simulink model "PART_5_COMBINED_HWY"  (R2025a)
settings: Solver=ode4  StartTime=0.0  StopTime=763  RelTol=1e-3
values from neighbouring files (symbols this model uses):
  Air_density = 1.225    [PART_5_CITY.m]    (also in PART_5_HWY.m; PART_5_SCO3.m; PART_5_US06_MODEL.m)
  Coefficient_of_rolling_resistance = 0.012    [PART_5_CITY.m]    (also in PART_5_HWY.m; PART_5_SCO3.m; PART_5_US06_MODEL.m)
  Drag_coefficient = 0.2    [PART_5_CITY.m]    (also in PART_5_HWY.m; PART_5_SCO3.m; PART_5_US06_MODEL.m)
  Driveline_model_spinloss = 6    [PART_5_CITY.m]    (also in PART_5_HWY.m; PART_5_SCO3.m; PART_5_US06_MODEL.m)
  energy_capacity = 12.6    [PART_5_CITY.m]    (also in PART_5_HWY.m; PART_5_SCO3.m; PART_5_US06_MODEL.m)
  Frontal_Area = 1.8    [PART_5_CITY.m]    (also in PART_5_HWY.m; PART_5_SCO3.m; PART_5_US06_MODEL.m)
  Gear_Ratio_g = 7    [PART_5_CITY.m]    (also in PART_5_HWY.m; PART_5_SCO3.m; PART_5_US06_MODEL.m)
  grade_angle = 15    [PART_5_CITY.m]    (also in PART_5_HWY.m; PART_5_SCO3.m; PART_5_US06_MODEL.m)
  Gravitational_force = 9.81    [PART_5_CITY.m]    (also in PART_5_HWY.m; PART_5_SCO3.m; PART_5_US06_MODEL.m)
  initial_soc = 0.95    [PART_5_CITY.m]    (also in PART_5_HWY.m; PART_5_SCO3.m; PART_5_US06_MODEL.m)
  MDL_brakesystem_friction = 0.45    [PART_5_CITY.m]    (also in PART_5_HWY.m; PART_5_SCO3.m; PART_5_US06_MODEL.m)
  MDL_brakesystem_regenerative_friction = 0.55    [PART_5_CITY.m]    (also in PART_5_HWY.m; PART_5_SCO3.m; PART_5_US06_MODEL.m)
  MDL_Brakingsystem_maximum_brakeforce = 10000    [PART_5_CITY.m]    (also in PART_5_HWY.m; PART_5_SCO3.m; PART_5_US06_MODEL.m)
  MDL_motormodel_Kc = 0.045257    [PART_5_CITY.m]    (also in PART_5_HWY.m; PART_5_SCO3.m; PART_5_US06_MODEL.m)
  MDL_motormodel_max_power_out = 100000    [PART_5_CITY.m]    (also in PART_5_HWY.m; PART_5_SCO3.m; PART_5_US06_MODEL.m)
  MDL_motormodel_maxtorque_out = 500    [PART_5_CITY.m]    (also in PART_5_HWY.m; PART_5_SCO3.m; PART_5_US06_MODEL.m)
  MotorModel_C = 628.3    [PART_5_CITY.m]    (also in PART_5_HWY.m; PART_5_SCO3.m; PART_5_US06_MODEL.m)
  MotorModel_ki = 0.016667    [PART_5_CITY.m]    (also in PART_5_HWY.m; PART_5_SCO3.m; PART_5_US06_MODEL.m)
  MotorModel_kw = 5.0664*10^-5    (= 5.0664e-05)    [PART_5_CITY.m]    (also in PART_5_HWY.m; PART_5_SCO3.m; PART_5_US06_MODEL.m)
  total_weight = 2154.6    [PART_5_CITY.m]    (also in PART_5_HWY.m; PART_5_SCO3.m; PART_5_US06_MODEL.m)
  wheel_radius_cal = 0.217    [PART_5_CITY.m]    (also in PART_5_HWY.m; PART_5_SCO3.m; PART_5_US06_MODEL.m)
undefined symbols (not defined in the file or in its folder): m, magnitude, s
libraries: simulink x5, aerolibconvert2 x4, slpidlib x1
settings Model: Creator=user  LastModifiedBy=user

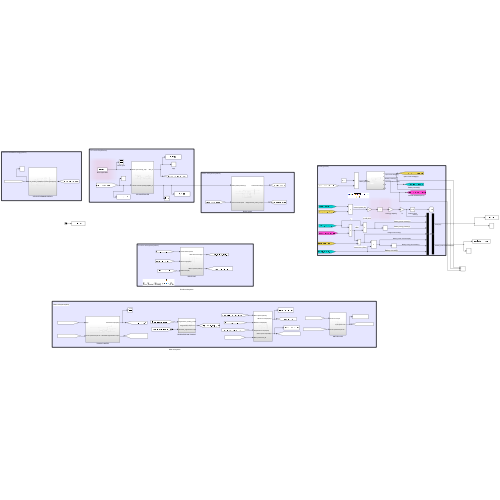
[thumbnail: Simulink's stored preview of the top-level diagram]
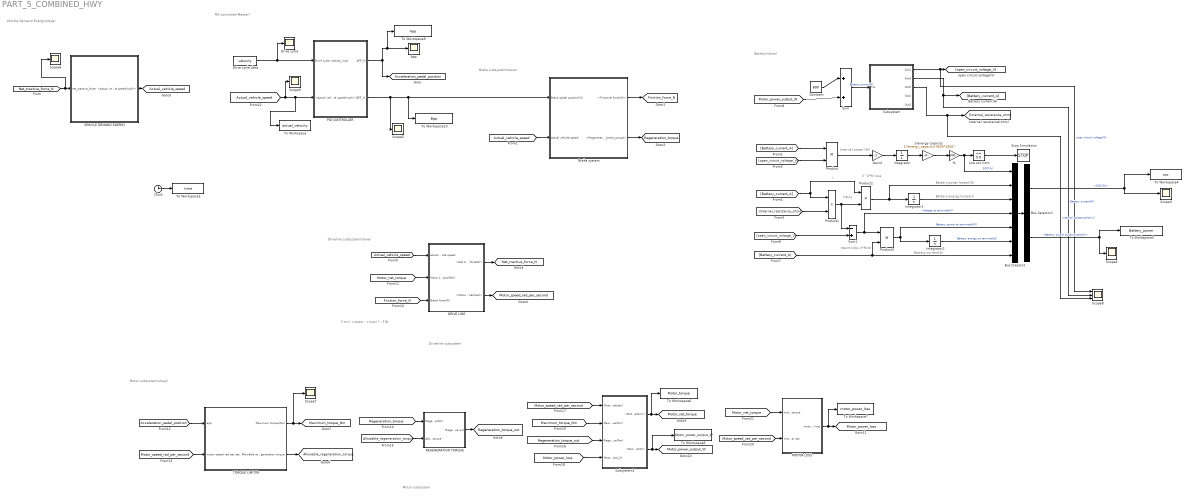
== system PART_5_COMBINED_HWY ==
  note: F tr=( τ motor - τ loss) * - F Br
  note: PID controller(Master)
  note: Driveline subsystem
  note: Vehicle Demand Energy(slave)
  note: Motor subsystem
  note: Driveline subsystem(slave)
  note: Brake subsystem(slave)
  note: Battery energy losses(J)
  note: (I^2*R) loss
  note: Battery power losses(W)
  note: Battery(slave)
  note: I*Rint
  note: Battery current(A)
  note: Internal power (W)
  note: I
  note: Motor subsystem(slave)
  note: Vterm=Voc-(I*Rint)
  % : Gain  Gain=100
  1/energy capacity : Gain  Gain=1/(energy_capacity*3600*1000)
  App : Scope
      settings: ActiveDisplayYMinimum=-0.92182  ActiveDisplayYMaximum=8.29642
  Brake system : Subsystem
  Bus Creator2 : BusCreator  Inputs=7
  Bus Selector1 : BusSelector  OutputSignals=SOC(%),Battery power at terminals(W)
  Clock : Clock
  Constant : Constant  Value=600
  DRIVE LINE : Subsystem
  Drive cycle : Scope
      settings: ActiveDisplayYMinimum=-10.0375  ActiveDisplayYMaximum=90.3375  DataLoggingVariableName=ScopeData12
  Drive cycle data : FromWorkspace  VariableName=velocity  SampleTime=0.1
  Gain4 : Gain  Gain=-1
  Integrator : Integrator  InitialCondition=energy_capacity*3600*1000*initial_soc
  Integrator1 : Integrator
  Integrator2 : Integrator
  Low soc limit : simulink/Logic and Bit Operations/Compare To Constant  relop=<=  const=5.0  OutDataTypeStr=boolean
  MOTOR LOSS : Subsystem
  PID CONTROLLER : Subsystem
  Product{,1..3} (4 alike) : Product
  REGENERATION TORQUE : Subsystem
  Scope{3..7,9} (6 alike) : Scope
      Scope3 settings: ActiveDisplayYMinimum=-1  ActiveDisplayYMaximum=1  DataLoggingVariableName=ScopeData13
      Scope4 settings: ActiveDisplayYMinimum=-68149.999999999942  ActiveDisplayYMaximum=119350.00000000003  DataLoggingVariableName=ScopeData14
      Scope5 settings: ActiveDisplayYMinimum=-1  ActiveDisplayYMaximum=1  DataLoggingVariableName=ScopeData6
      Scope6 settings: ActiveDisplayYMinimum=-11875  ActiveDisplayYMaximum=6875  DataLoggingVariableName=ScopeData15
      Scope7 settings: ActiveDisplayYMinimum=-1  ActiveDisplayYMaximum=1  DataLoggingVariableName=ScopeData16
      Scope9 settings: ActiveDisplayYMinimum=-1  ActiveDisplayYMaximum=1  DataLoggingVariableName=ScopeData17
  Scope8 : Scope  NumInputPorts=3
      settings: ActiveDisplayYMinimum=-1  ActiveDisplayYMaximum=1  DataLoggingVariableName=ScopeData9
  Stop Simulation : Stop
  Subsystem : Subsystem
  Subsystem1 : Subsystem
  Sum : Sum  Inputs=|++
  Sum1 : Sum  Inputs=-+
  TORQUE LIMITER : Subsystem
  To Workspace : ToWorkspace  VariableName=actual_velocity  SampleTime=-1
      settings: Save2DSignal=2-D array (concatenate along first dimension)
  To Workspace1 : ToWorkspace  VariableName=time  SampleTime=-1
      settings: Save2DSignal=2-D array (concatenate along first dimension)
  To Workspace10 : ToWorkspace  VariableName=Bpp  SampleTime=-1
      settings: Save2DSignal=2-D array (concatenate along first dimension)
  To Workspace4 : ToWorkspace  VariableName=soc  SampleTime=-1
      settings: Save2DSignal=2-D array (concatenate along first dimension)
  To Workspace5 : ToWorkspace  VariableName=Battery_power  SampleTime=-1
      settings: Save2DSignal=2-D array (concatenate along first dimension)
  To Workspace6 : ToWorkspace  VariableName=Motor_torque  SampleTime=-1
      settings: Save2DSignal=2-D array (concatenate along first dimension)
  To Workspace7 : ToWorkspace  VariableName=motor_power_loss  SampleTime=-1
      settings: Save2DSignal=2-D array (concatenate along first dimension)
  To Workspace8 : ToWorkspace  VariableName=Motor_power_output_W  SampleTime=-1
      settings: Save2DSignal=2-D array (concatenate along first dimension)
  To Workspace9 : ToWorkspace  VariableName=App  SampleTime=-1
      settings: Save2DSignal=2-D array (concatenate along first dimension)
  VEHICLE DEMAND ENERGY : Subsystem
  tag scope: Acceleration_pedal_position=global, Actual_vehicle_speed=global, Allowable_regeneration_torque=global, Friction_force_N=global, Maximum_torque_Nm=global, Motor_net_torque=global, Motor_power_loss=global, Motor_power_output_W=global, Motor_speed_rad_per_second=global, Net_tractive_force_N=global, Regeneration_torque=global, Regeneration_torque_out=global
  wires:
  [Internal_resistance_ohm] -> Product1/2
  Integrator2/1 -> Bus Creator2/6  "Battery energy at terminals(J)"
  Subsystem/2(Out4) -> Scope8/2, [Battery_current_A]  "Battery current(A)"
  [Maximum_torque_Nm] -> Subsystem1/2(Maximum torque(Nm))
  [Battery_current_A] -> Product/1
  DRIVE LINE/2(<Motor speed (rad/sec)>) -> [Motor_speed_rad_per_second]
  [Friction_force_N] -> DRIVE LINE/3(Brake force(N))
  [Motor_net_torque] -> MOTOR LOSS/1(motor net torque)
  %/1 -> Bus Creator2/1, Low soc limit/1  "SOC(%)"
  Subsystem/3(Out5) -> Scope8/3, [Internal_resistance_ohm]  "Internal resistance(ohm)"
  Drive cycle data/1 -> Drive cycle/1, PID CONTROLLER/1(Drive cycle velocity_mph)
  Subsystem/1(Out1) -> Scope8/1, [open_circuit_voltage_V]  "open circuit voltage(V)"
  Subsystem1/1(<Motor net torque(Nm)>) -> To Workspace6/1, [Motor_net_torque]
  [Actual_vehicle_speed] -> DRIVE LINE/1(actual vehicle speed)
  [Motor_power_output_W] -> Sum/2
  Bus Selector1/1 -> To Workspace4/1, Scope3/1  "<SOC(%)>"
  [Net_tractive_force_N] -> Scope6/1, VEHICLE DEMAND ENERGY/1(net_tractive_force)
  Product/1 -> Gain4/1
  Low soc limit/1 -> Stop Simulation/1
  [Motor_speed_rad_per_second] -> Subsystem1/1(Motor speed (rad/sec))
  DRIVE LINE/1(<Net tractive force(N)>) -> [Net_tractive_force_N]
  [Motor_speed_rad_per_second] -> MOTOR LOSS/2(motor speed rad per sec)
  Sum/1 -> Subsystem/1(In1)  "Battery power(W)"
  [Regeneration_torque] -> REGENERATION TORQUE/1(Regeneration_braking_torque(Nm))
  Product3/1 -> Integrator2/1, Bus Creator2/5  "Battery power at terminals(W)"
  Product1/1 -> Sum1/1, Product2/2
  [Actual_vehicle_speed] -> Scope9/1, To Workspace/1, PID CONTROLLER/2(<Actual vehicle speed(mph)>)
  Brake system/2(<Regenerative_brake_torque>) -> [Regeneration_torque]
  REGENERATION TORQUE/1(Regeneration torque out) -> [Regeneration_torque_out]
  [Motor_net_torque] -> DRIVE LINE/2(Motor torque(Nm))
  Subsystem1/2(<Motor power output(W)>) -> To Workspace8/1, [Motor_power_output_W]
  [Regeneration_torque_out] -> Subsystem1/3(Regeneration torque(Nm))
  Integrator/1 -> 1/energy capacity/1
  [Allowable_regeneration_torque] -> REGENERATION TORQUE/2(Allowable_regeneration torque)
  [Battery_current_A] -> Product3/2, Bus Creator2/7
  [Motor_speed_rad_per_second] -> TORQUE LIMITER/2(motor speed rad per sec)
  Sum1/1 -> Product3/1, Bus Creator2/4  "Voltage at terminals(V)"
  MOTOR LOSS/1(motor power loss) -> To Workspace7/1, [Motor_power_loss]
  [Acceleration_pedal_position] -> TORQUE LIMITER/1(app)
  PID CONTROLLER/2(BPP_%) -> To Workspace10/1, Brake system/1(Brake pedal position(%)), Scope5/1
  Brake system/1(<Frictional force(N)>) -> [Friction_force_N]
  PID CONTROLLER/1(APP_%) -> To Workspace9/1, App/1, [Acceleration_pedal_position]
  Product2/1 -> Bus Creator2/2, Integrator1/1
  Bus Selector1/2 -> Scope4/1, To Workspace5/1  "<Battery power at terminals(W)>"
  Integrator1/1 -> Bus Creator2/3
  [Motor_power_loss] -> Subsystem1/4(Motor power loss_W)
  TORQUE LIMITER/1(Maximum torque(Nm)) -> Scope7/1, [Maximum_torque_Nm]
  1/energy capacity/1 -> %/1
  Constant/1 -> Sum/1
  TORQUE LIMITER/2(Allowable regeneration torque) -> [Allowable_regeneration_torque]
  [open_circuit_voltage_V] -> Sum1/2
  Gain4/1 -> Integrator/1
  Clock/1 -> To Workspace1/1
  Bus Creator2/1 -> Bus Selector1/1
  VEHICLE DEMAND ENERGY/1(<Actual vehicle speed(mph)>) -> [Actual_vehicle_speed]
  [open_circuit_voltage_V] -> Product/2
  [Actual_vehicle_speed] -> Brake system/2(Actual vehicle speed)
  [Battery_current_A] -> Product2/1, Product1/1

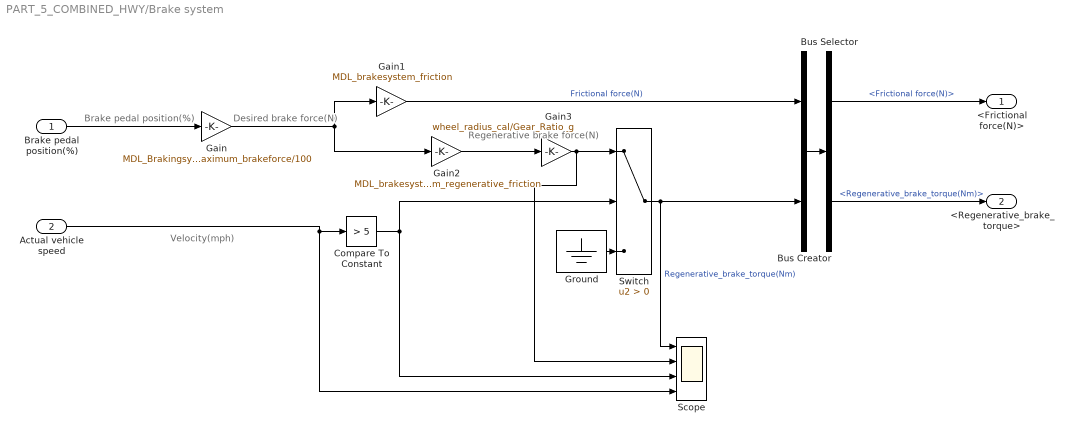
== system PART_5_COMBINED_HWY/Brake system ==
  note: Desired brake force(N)
  note: Brake pedal position(%)
  note: Velocity(mph)
  note: Regenerative
      | brake force(N)
  Brake pedal position(%) : Inport
  Actual vehicle speed : Inport  Port=2
  Bus Creator : BusCreator  Inputs=2
  Bus Selector : BusSelector  OutputSignals=Frictional force(N),Regenerative_brake_torque(Nm)
  Compare To Constant : simulink/Logic and Bit Operations/Compare To Constant  relop=>  const=5  OutDataTypeStr=boolean
  Gain : Gain  Gain=MDL_Brakingsystem_maximum_brakeforce/100
  Gain1 : Gain  Gain=MDL_brakesystem_friction
  Gain2 : Gain  Gain=MDL_brakesystem_regenerative_friction
  Gain3 : Gain  Gain=wheel_radius_cal/Gear_Ratio_g
  Ground : Ground
  Scope : Scope  NumInputPorts=4
      settings: ActiveDisplayYMinimum=-1  ActiveDisplayYMaximum=1  DataLoggingVariableName=ScopeData3
  Switch : Switch  Criteria=u2 > Threshold  SaturateOnIntegerOverflow=off  InputSameDT=off
  <Frictional force(N)> : Outport
  <Regenerative_brake_torque> : Outport  Port=2
  wires:
  Gain2/1 -> Gain3/1
  Switch/1 -> Bus Creator/2, Scope/1  "Regenerative_brake_torque(Nm)"
  Bus Creator/1 -> Bus Selector/1
  Gain1/1 -> Bus Creator/1  "Frictional force(N)"
  Compare To Constant/1 -> Scope/3, Switch/2
  Gain3/1 -> Scope/2, Switch/1
  Ground/1 -> Switch/3
  Gain/1 -> Gain2/1, Gain1/1
  Actual vehicle speed/1 -> Scope/4, Compare To Constant/1
  Bus Selector/2 -> <Regenerative_brake_torque>/1  "<Regenerative_brake_torque(Nm)>"
  Brake pedal position(%)/1 -> Gain/1
  Bus Selector/1 -> <Frictional force(N)>/1  "<Frictional force(N)>"

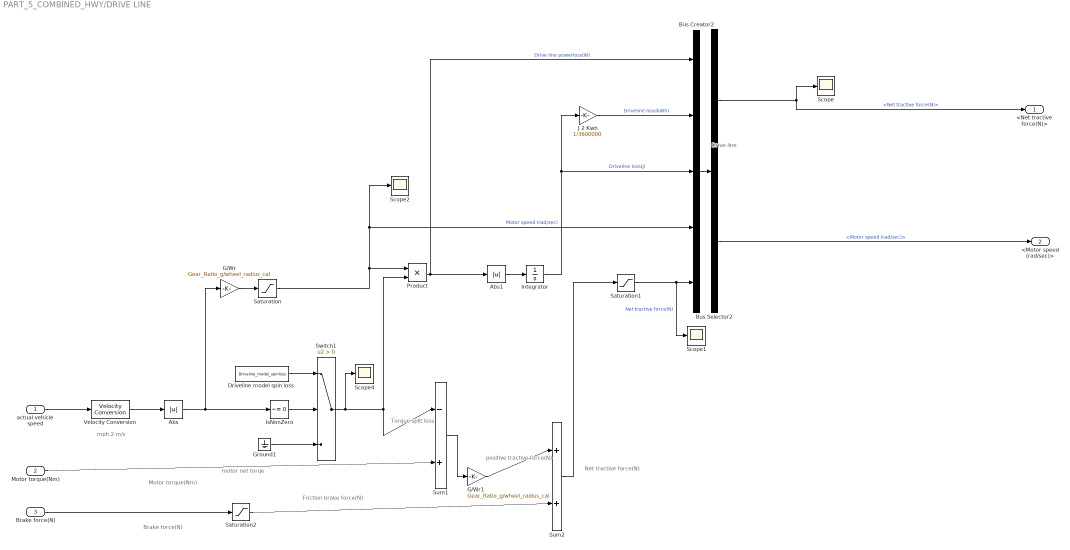
== system PART_5_COMBINED_HWY/DRIVE LINE ==
  note: Drive line
  note: Friction brake force(N)
  note: Net tractive force(N)
  note: motor net torqe
  note: positive tractive force(N)
  note: mph 2 m/s
  note: Motor torque(Nm)
  note: Torque split
      |  loss
  note: Brake force(N)
  actual vehicle speed : Inport
  Motor torque(Nm) : Inport  Port=2
  Brake force(N) : Inport  Port=3
  Abs : Abs  SaturateOnIntegerOverflow=off
  Abs1 : Abs  SaturateOnIntegerOverflow=off
  Bus Creator2 : BusCreator  Inputs=5
  Bus Selector2 : BusSelector  OutputSignals=Net tractive force(N),Motor speed (rad/sec)
  Driveline model spin loss : Constant  Value=Driveline_model_spinloss  OutDataTypeStr=double
  G/Wr : Gain  Gain=Gear_Ratio_g/wheel_radius_cal
  G/Wr1 : Gain  Gain=Gear_Ratio_g/wheel_radius_cal
  Ground1 : Ground
  Integrator : Integrator
  IsNonZero : simulink/Logic and Bit Operations/Compare To Zero  relop=~=  OutDataTypeStr=boolean
  J 2 Kwh : Gain  Gain=1/3600000
  Product : Product
  Saturation : Saturate  UpperLimit=inf  LowerLimit=.00001
  Saturation1 : Saturate  UpperLimit=5000  LowerLimit=-10000  OutDataTypeStr=double
  Saturation2 : Saturate  UpperLimit=0  LowerLimit=-10000
  Scope{,1..2,4} (4 alike) : Scope
      Scope settings: ActiveDisplayYMinimum=-1  ActiveDisplayYMaximum=1
      Scope1 settings: ActiveDisplayYMinimum=-10214.22916  ActiveDisplayYMaximum=10023.80324  DataLoggingVariableName=ScopeData3
      Scope2 settings: ActiveDisplayYMinimum=-7.75811  ActiveDisplayYMaximum=69.82309  DataLoggingVariableName=ScopeData4
      Scope4 settings: ActiveDisplayYMinimum=-0.75  ActiveDisplayYMaximum=6.75  DataLoggingVariableName=ScopeData11
  Sum1 : Sum  Inputs=|-+
  Sum2 : Sum  Inputs=|++
  Switch1 : Switch  Criteria=u2 > Threshold  OutDataTypeStr=double  SaturateOnIntegerOverflow=off  InputSameDT=off
  Velocity Conversion : aerolibconvert2/Velocity Conversion  IU=mph  OU=m/s
  <Net tractive force(N)> : Outport
  <Motor speed (rad/sec)> : Outport  Port=2
  wires:
  Abs/1 -> IsNonZero/1, G/Wr/1
  Saturation/1 -> Bus Creator2/4, Scope2/1, Product/1  "Motor speed (rad/sec)"
  Abs1/1 -> Integrator/1
  Switch1/1 -> Product/2, Sum1/1, Scope4/1
  Sum2/1 -> Saturation1/1
  Ground1/1 -> Switch1/3
  Sum1/1 -> G/Wr1/1
  G/Wr1/1 -> Sum2/1
  Saturation1/1 -> Scope1/1, Bus Creator2/5  "Net tractive force(N)"
  Product/1 -> Bus Creator2/1, Abs1/1  "Drive line powerloss(W)"
  Integrator/1 -> J 2 Kwh/1, Bus Creator2/3  "Driveline loss(J)"
  G/Wr/1 -> Saturation/1
  J 2 Kwh/1 -> Bus Creator2/2  "Driveline loss(kWh)"
  actual vehicle speed/1 -> Velocity Conversion/1
  Bus Selector2/2 -> <Motor speed (rad/sec)>/1  "<Motor speed (rad/sec)>"
  IsNonZero/1 -> Switch1/2
  Velocity Conversion/1 -> Abs/1
  Bus Creator2/1 -> Bus Selector2/1
  Saturation2/1 -> Sum2/2
  Motor torque(Nm)/1 -> Sum1/2
  Bus Selector2/1 -> Scope/1, <Net tractive force(N)>/1  "<Net tractive force(N)>"
  Brake force(N)/1 -> Saturation2/1
  Driveline model spin loss/1 -> Switch1/1

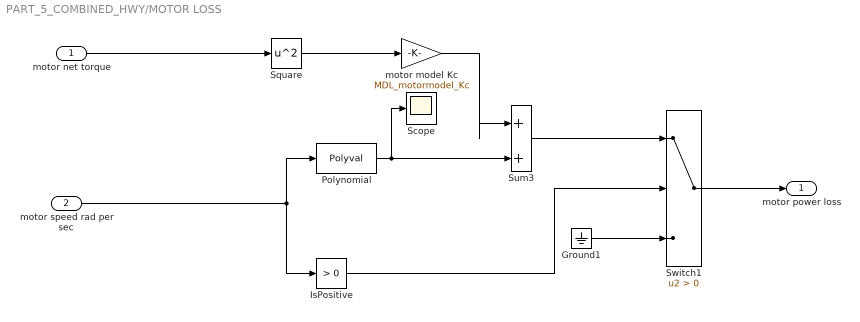
== system PART_5_COMBINED_HWY/MOTOR LOSS ==
  motor net torque : Inport
  motor speed rad per sec : Inport  Port=2
  Ground1 : Ground
  IsPositive : simulink/Logic and Bit Operations/Compare To Zero  relop=>  OutDataTypeStr=boolean
  Polynomial : Polyval  Coefs=[MotorModel_kw,0,MotorModel_ki,MotorModel_C]
  Scope : Scope
      settings: ActiveDisplayYMinimum=583.90938  ActiveDisplayYMaximum=1027.81559  DataLoggingVariableName=ScopeData5
  Square : Math  Operator=square
  Sum3 : Sum  Inputs=|++
  Switch1 : Switch  Criteria=u2 > Threshold  OutDataTypeStr=double  SaturateOnIntegerOverflow=off  InputSameDT=off
  motor model Kc : Gain  Gain=MDL_motormodel_Kc
  motor power loss : Outport
  wires:
  Polynomial/1 -> Scope/1, Sum3/2
  Sum3/1 -> Switch1/1
  Square/1 -> motor model Kc/1
  Ground1/1 -> Switch1/3
  motor model Kc/1 -> Sum3/1
  IsPositive/1 -> Switch1/2
  Switch1/1 -> motor power loss/1
  motor net torque/1 -> Square/1
  motor speed rad per sec/1 -> Polynomial/1, IsPositive/1

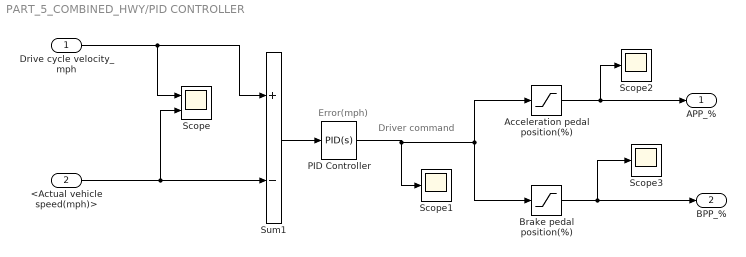
== system PART_5_COMBINED_HWY/PID CONTROLLER ==
  note: Driver command
  note: Error(mph)
  Drive cycle velocity_mph : Inport
  <Actual vehicle speed(mph)> : Inport  Port=2
  Acceleration pedal position(%) : Saturate  UpperLimit=100  LowerLimit=0  LinearizeAsGain=off  ZeroCross=off  OutDataTypeStr=double
  Brake pedal position(%) : Saturate  UpperLimit=0  LowerLimit=-100  LinearizeAsGain=off  ZeroCross=off  OutDataTypeStr=double
  PID Controller : slpidlib/PID Controller  Controller=PID  Form=Parallel  TimeDomain=Continuous-time  UseExternalTs=off  SampleTime=-1  IntegratorMethod=Forward Euler  FilterMethod=Forward Euler  ControllerParametersSource=internal  P=250  I=50  UseKiTs=off  D=0  UseExternalDerivativeSource=off  N=10  UseFilter=on  TunerSelectOption=Transfer Function Based (PID Tuner App)  InitialConditionSource=internal  InitialConditionForIntegrator=0  InitialConditionForFilter=0  DifferentiatorICPrevScaledInput=0  ExternalReset=none  TrackingMode=off  Kt=1  LimitOutput=off  SatLimitsSource=internal  UpperSaturationLimit=inf  LowerSaturationLimit=-inf  LinearizeAsGain=off  AntiWindupMode=none  Kb=1  LimitIntegrator=off  UpperIntegratorSaturationLimit=inf  LowerIntegratorSaturationLimit=-inf  POutMin=[]  POutMax=[]  IOutMin=[]  IOutMax=[]  DOutMin=[]  DOutMax=[]  NOutMin=[]  NOutMax=[]  SumOutMin=[]  SumOutMax=[]  SaturationOutMin=[]  SaturationOutMax=[]  PParamMin=[]  PParamMax=[]  IParamMin=[]  IParamMax=[]  DParamMin=[]  DParamMax=[]  NParamMin=[]  NParamMax=[]  KbParamMin=[]  KbParamMax=[]  KtParamMin=[]  KtParamMax=[]  KbOutMin=[]  KbOutMax=[]  KtOutMin=[]  KtOutMax=[]  IntegratorOutMin=[]  IntegratorOutMax=[]  FilterOutMin=[]  FilterOutMax=[]  SumI1OutMin=[]  SumI1OutMax=[]  SumI2OutMin=[]  SumI2OutMax=[]  SumI3OutMin=[]  SumI3OutMax=[]  SumI4OutMin=[]  SumI4OutMax=[]  SumDOutMin=[]  SumDOutMax=[]  DifferentiatorOutMin=[]  DifferentiatorOutMax=[]  FilterDiffOutCoefMin=[]  FilterDiffOutCoefMax=[]  ReciprocalOutMin=[]  ReciprocalOutMax=[]  SumDenOutMin=[]  SumDenOutMax=[]  SumNumOutMin=[]  SumNumOutMax=[]  DivideOutMin=[]  DivideOutMax=[]  UdiffTsProdOutMin=[]  UdiffTsProdOutMax=[]  NTsProdOutMin=[]  NTsProdOutMax=[]  UintegralTsProdOutMin=[]  UintegralTsProdOutMax=[]  UngainTsProdOutMin=[]  UngainTsProdOutMax=[]  ClampingZeroOutDataTypeStr=Inherit: Inherit via back propagation  ClampingZeroOutMin=[]  ClampingZeroOutMax=[]  FilterDenConstantOutDataTypeStr=Inherit: Inherit via back propagation  FilterDenConstantOutMin=[]  FilterDenConstantOutMax=[]  PCopyOutDataTypeStr=Inherit: Inherit via back propagation  PCopyOutMin=[]  PCopyOutMax=[]  NCopyOutDataTypeStr=Inherit: Inherit via back propagation  NCopyOutMin=[]  NCopyOutMax=[]  IntegratorContinuousStateAttributes=''  IntegratorStateMustResolveToSignalObject=off  IntegratorRTWStateStorageClass=Auto  FilterContinuousStateAttributes=''  FilterStateMustResolveToSignalObject=off  FilterRTWStateStorageClass=Auto  ParallelPVariant=InternalParameters  IdealPVariant=Disabled  IVariant=InternalParameters  DVariant=InternalParameters  IntegratorVariant=Continuous  SatVariant=Disabled  AWVariant=Passthrough  PCopyVariant=Disabled  TRVariant=Disabled  FdbkBlocksVariant=Forward  IdealPFdbkVariant=Disabled  SatFdbkVariant=Disabled  DerivativeFilterVariant=ContFilter  NVariant=InternalParameters  NCopyVariant=Disabled  FilterICVariant=InternalICsFilter  IntegratorICVariant=InternalICs  ExternalResetVariant=Disabled  TRSumVariant=Passthrough  SumFdbkVariant=Disabled  SumVariant=Sum_PID  TsampFilterVariant=InternalTs  TsampNgainVariant=Passthrough  TsampIntegralVariant=Disabled_SignalSpec  ExternalSaturationOutDataTypeStr=Inherit: Same as second input  DerivativeSourceVariant=ErrorSignal  PreIntVariant=InternalPreInt
  Scope : Scope  NumInputPorts=2
      settings: ActiveDisplayYMinimum=-1  ActiveDisplayYMaximum=1
  Scope1 : Scope
      settings: ActiveDisplayYMinimum=-1  ActiveDisplayYMaximum=1
  Scope2 : Scope
      settings: ActiveDisplayYMinimum=-1  ActiveDisplayYMaximum=1  DataLoggingVariableName=ScopeData10
  Scope3 : Scope
      settings: ActiveDisplayYMinimum=-1  ActiveDisplayYMaximum=1
  Sum1 : Sum  Inputs=+-
  APP_% : Outport
  BPP_% : Outport  Port=2
  wires:
  Acceleration pedal position(%)/1 -> Scope2/1, APP_%/1
  <Actual vehicle speed(mph)>/1 -> Scope/2, Sum1/2
  Drive cycle velocity_mph/1 -> Sum1/1, Scope/1
  Sum1/1 -> PID Controller/1
  PID Controller/1 -> Scope1/1, Brake pedal position(%)/1, Acceleration pedal position(%)/1
  Brake pedal position(%)/1 -> BPP_%/1, Scope3/1

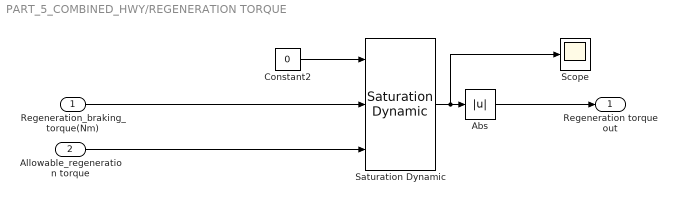
== system PART_5_COMBINED_HWY/REGENERATION TORQUE ==
  Regeneration_braking_torque(Nm) : Inport
  Allowable_regeneration torque : Inport  Port=2
  Abs : Abs  SaturateOnIntegerOverflow=off
  Constant2 : Constant  Value=0
  Saturation Dynamic : simulink/Discontinuities/Saturation Dynamic  OutMin=[]  OutMax=[]  OutDataTypeStr=Inherit: Same as second input  OutDataType=fixdt(1, 16)  OutScaling=2^-10  DoSatur=off
  Scope : Scope
      settings: ActiveDisplayYMinimum=-191.8125  ActiveDisplayYMaximum=21.3125  DataLoggingVariableName=ScopeData2
  Regeneration torque out : Outport
  wires:
  Saturation Dynamic/1 -> Scope/1, Abs/1
  Abs/1 -> Regeneration torque out/1
  Constant2/1 -> Saturation Dynamic/1
  Regeneration_braking_torque(Nm)/1 -> Saturation Dynamic/2
  Allowable_regeneration torque/1 -> Saturation Dynamic/3

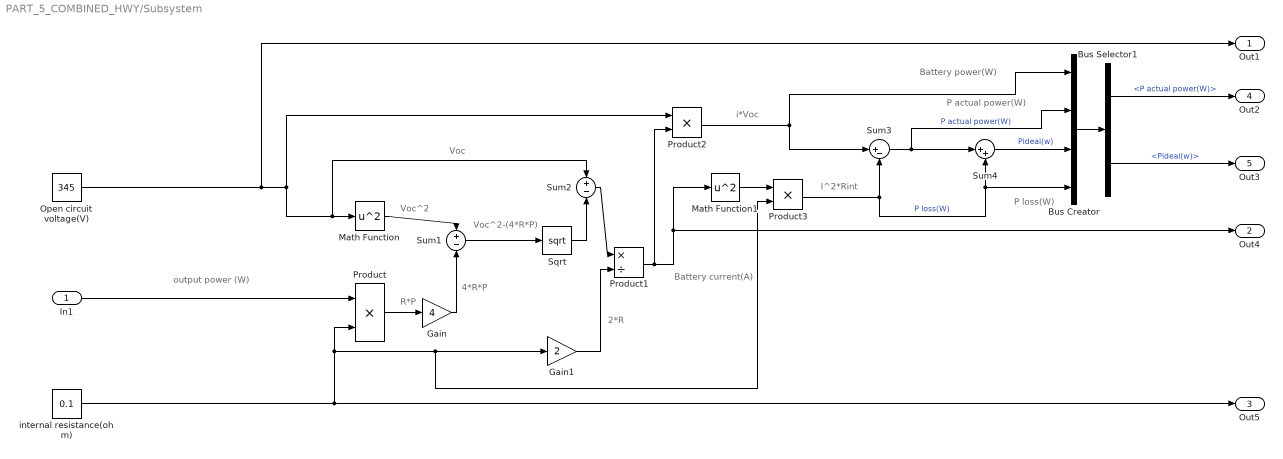
== system PART_5_COMBINED_HWY/Subsystem ==
  note: Voc^2
  note: 4*R*P
  note: 2*R
  note: Voc
  note: output power (W)
  note: Battery current(A)
  note: i*Voc
  note: P loss(W)
  note: R*P
  note: I^2*Rint
  note: Battery power(W)
  note: P actual power(W)
  note: Voc^2-(4*R*P)
  In1 : Inport
  Bus Creator : BusCreator  Inputs=4
  Bus Selector1 : BusSelector  OutputSignals=P actual power(W),Pideal(w)
  Gain : Gain  Gain=4
  Gain1 : Gain  Gain=2
  Math Function : Math  Operator=square
  Math Function1 : Math  Operator=square
  Open circuit voltage(V) : Constant  Value=345
  Product : Product
  Product1 : Product  Inputs=*/
  Product2 : Product
  Product3 : Product
  Sqrt : Sqrt
  Sum1 : Sum  Inputs=+-
  Sum2 : Sum  Inputs=+-
  Sum3 : Sum  Inputs=|+-
  Sum4 : Sum  Inputs=|++
  internal resistance(ohm) : Constant  Value=0.1
  Out1 : Outport
  Out4 : Outport  Port=2
  Out5 : Outport  Port=3
  Out2 : Outport  Port=4
  Out3 : Outport  Port=5
  wires:
  Open circuit voltage(V)/1 -> Out1/1, Sum2/1, Math Function/1, Product2/1
  internal resistance(ohm)/1 -> Product/2, Product3/2, Gain1/1, Out5/1
  Math Function1/1 -> Product3/1
  Bus Creator/1 -> Bus Selector1/1
  Product1/1 -> Product2/2, Out4/1, Math Function1/1
  Sum3/1 -> Bus Creator/2, Sum4/1  "P actual power(W)"
  Gain1/1 -> Product1/2
  Product2/1 -> Bus Creator/1, Sum3/1
  Sum4/1 -> Bus Creator/3  "Pideal(w)"
  Bus Selector1/1 -> Out2/1  "<P actual power(W)>"
  Product3/1 -> Sum4/2, Bus Creator/4, Sum3/2  "P loss(W)"
  Gain/1 -> Sum1/2
  Product/1 -> Gain/1
  Sqrt/1 -> Sum2/2
  Sum2/1 -> Product1/1
  Math Function/1 -> Sum1/1
  Sum1/1 -> Sqrt/1
  In1/1 -> Product/1
  Bus Selector1/2 -> Out3/1  "<Pideal(w)>"

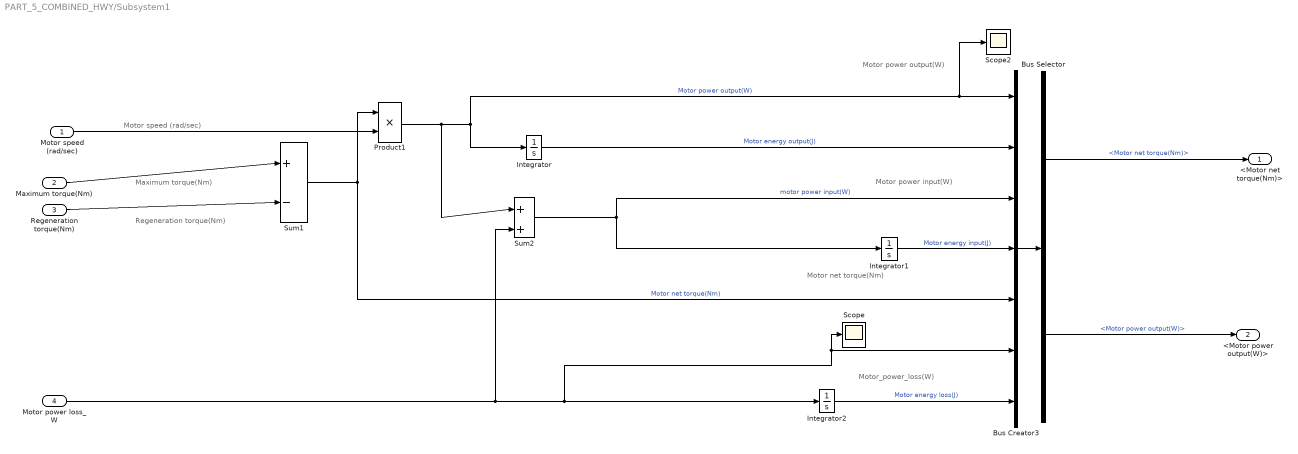
== system PART_5_COMBINED_HWY/Subsystem1 ==
  note: Motor speed (rad/sec)
  note: Regeneration torque(Nm)
  note: Maximum torque(Nm)
  note: Motor_power_loss(W)
  note: Motor net torque(Nm)
  note: Motor power output(W)
  note: Motor power input(W)
  Motor speed (rad/sec) : Inport
  Maximum torque(Nm) : Inport  Port=2
  Regeneration torque(Nm) : Inport  Port=3
  Motor power loss_W : Inport  Port=4
  Bus Creator3 : BusCreator  Inputs=7
  Bus Selector : BusSelector  OutputSignals=Motor net torque(Nm),Motor power output(W)
  Integrator : Integrator
  Integrator1 : Integrator
  Integrator2 : Integrator
  Product1 : Product
  Scope : Scope
      settings: ActiveDisplayYMinimum=-836.47395  ActiveDisplayYMaximum=13811.26552  DataLoggingVariableName=ScopeData2
  Scope2 : Scope
      settings: ActiveDisplayYMinimum=-879.44705  ActiveDisplayYMaximum=7915.02342  DataLoggingVariableName=ScopeData7
  Sum1 : Sum  Inputs=|+-
  Sum2 : Sum  Inputs=|++
  <Motor net torque(Nm)> : Outport
  <Motor power output(W)> : Outport  Port=2
  wires:
  Integrator/1 -> Bus Creator3/2  "Motor energy output(J)"
  Bus Creator3/1 -> Bus Selector/1
  Integrator2/1 -> Bus Creator3/7  "Motor energy loss(J)"
  Product1/1 -> Sum2/1, Integrator/1, Scope2/1, Bus Creator3/1  "Motor power output(W)"
  Integrator1/1 -> Bus Creator3/4  "Motor energy input(J)"
  Sum2/1 -> Bus Creator3/3, Integrator1/1  "motor power input(W)"
  Bus Selector/1 -> <Motor net torque(Nm)>/1  "<Motor net torque(Nm)>"
  Motor power loss_W/1 -> Integrator2/1, Scope/1, Bus Creator3/6, Sum2/2
  Sum1/1 -> Bus Creator3/5, Product1/1  "Motor net torque(Nm)"
  Motor speed (rad/sec)/1 -> Product1/2
  Bus Selector/2 -> <Motor power output(W)>/1  "<Motor power output(W)>"
  Maximum torque(Nm)/1 -> Sum1/1
  Regeneration torque(Nm)/1 -> Sum1/2

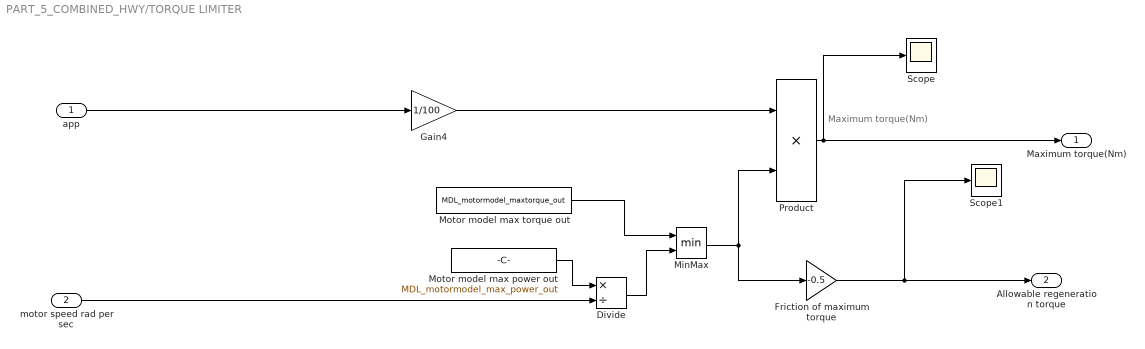
== system PART_5_COMBINED_HWY/TORQUE LIMITER ==
  note: Maximum torque(Nm)
  app : Inport
  motor speed rad per sec : Inport  Port=2
  Divide : Product  Inputs=*/
  Friction of maximum torque : Gain  Gain=-0.5
  Gain4 : Gain  Gain=1/100
  MinMax : MinMax  Inputs=2
  Motor model max power out : Constant  Value=MDL_motormodel_max_power_out  OutDataTypeStr=double
  Motor model max torque out : Constant  Value=MDL_motormodel_maxtorque_out  OutDataTypeStr=double
  Product : Product
  Scope : Scope
      settings: ActiveDisplayYMinimum=-62.5  ActiveDisplayYMaximum=562.5
  Scope1 : Scope
      settings: ActiveDisplayYMinimum=-350  ActiveDisplayYMaximum=-150  DataLoggingVariableName=ScopeData8
  Maximum torque(Nm) : Outport
  Allowable regeneration torque : Outport  Port=2
  wires:
  Divide/1 -> MinMax/2
  app/1 -> Gain4/1
  Gain4/1 -> Product/1
  motor speed rad per sec/1 -> Divide/2
  MinMax/1 -> Friction of maximum torque/1, Product/2
  Friction of maximum torque/1 -> Scope1/1, Allowable regeneration torque/1
  Product/1 -> Maximum torque(Nm)/1, Scope/1
  Motor model max torque out/1 -> MinMax/1
  Motor model max power out/1 -> Divide/1

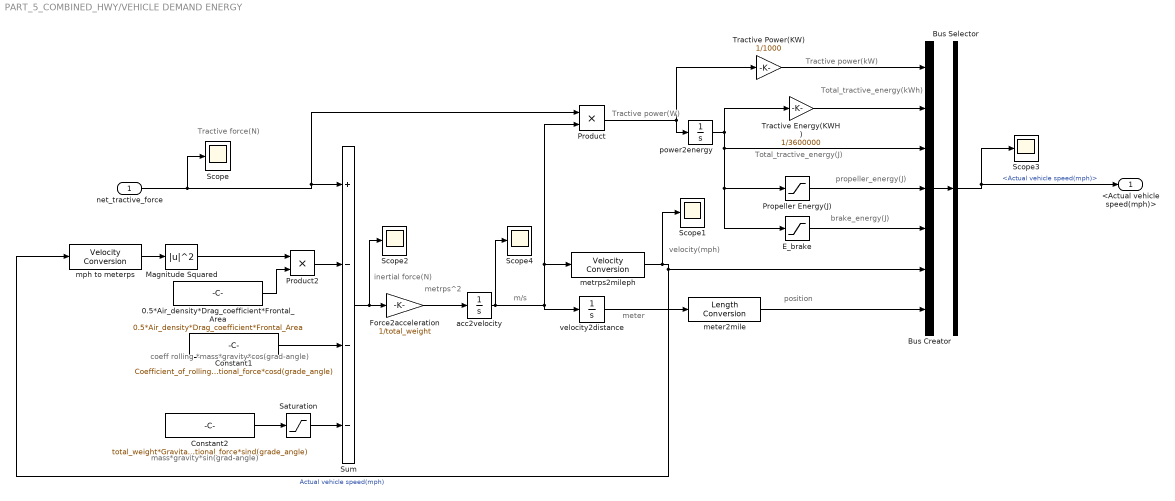
== system PART_5_COMBINED_HWY/VEHICLE DEMAND ENERGY ==
  note: Tractive force(N)
  note: mass*gravity*sin(grad-angle)
  note: metrps^2
  note: inertial force(N)
  note: Tractive power(W)
  note: velocity(mph)
  note: Total_tractive_energy(kWh)
  note: meter
  note: Total_tractive_energy(J)
  note: position
  note: m/s
  note: coeff rolling *mass*gravity*cos(grad-angle)
  note: brake_energy(J)
  note: propeller_energy(J)
  note: Tractive power(kW)
  net_tractive_force : Inport
  "   acc2velocity" : Integrator
  0.5*Air_density*Drag_coefficient*Frontal_Area : Constant  Value=0.5*Air_density*Drag_coefficient*Frontal_Area  OutDataTypeStr=double
  Bus Creator : BusCreator  Inputs=7
  Bus Selector : BusSelector  OutputSignals=Actual vehicle speed(mph)
  Constant1 : Constant  Value=Coefficient_of_rolling_resistance*total_weight*Gravitational_force*cosd(grade_angle)  OutDataTypeStr=double
  Constant2 : Constant  Value=total_weight*Gravitational_force*sind(grade_angle)  VectorParams1D=off  OutDataTypeStr=double
  E_brake : Saturate  UpperLimit=0  LowerLimit=-100
  "Force2acceleration   " : Gain  Gain=1/total_weight  ParamDataTypeStr=double  OutDataTypeStr=double
  Magnitude Squared : Math  Operator=magnitude^2  OutputSignalType=real  OutDataTypeStr=double
  Product : Product  OutDataTypeStr=double
  Product2 : Product
  Propeller Energy(J) : Saturate  UpperLimit=100  LowerLimit=0
  Saturation : Saturate  UpperLimit=244  LowerLimit=0
  Scope{,1..4} (5 alike) : Scope
      Scope settings: ActiveDisplayYMinimum=-7446.99841  ActiveDisplayYMaximum=5646.11287
      Scope1 settings: ActiveDisplayYMinimum=-5.60777  ActiveDisplayYMaximum=48.04799
      Scope2 settings: ActiveDisplayYMinimum=-7446.99841  ActiveDisplayYMaximum=5646.11287  DataLoggingVariableName=ScopeData2
      Scope3 settings: ActiveDisplayYMinimum=-10.04048  ActiveDisplayYMaximum=90.3643
      Scope4 settings: ActiveDisplayYMinimum=-2.5069  ActiveDisplayYMaximum=21.47937  DataLoggingVariableName=ScopeData3
  Sum : Sum  Inputs=+---  OutDataTypeStr=double  AccumDataTypeStr=double
  Tractive Energy(KWH) : Gain  Gain=1/3600000
  Tractive Power(KW) : Gain  Gain=1/1000
  meter2mile : aerolibconvert2/Length Conversion  IU=m  OU=mi
  metrps2mileph : aerolibconvert2/Velocity Conversion  IU=m/s  OU=mph
  mph to meterps : aerolibconvert2/Velocity Conversion  IU=mph  OU=m/s
  power2energy : Integrator
  velocity2distance : Integrator
  <Actual vehicle speed(mph)> : Outport
  wires:
  E_brake/1 -> Bus Creator/5
  power2energy/1 -> Bus Creator/3, E_brake/1, Propeller Energy(J)/1, Tractive Energy(KWH)/1
  Product/1 -> power2energy/1, Tractive Power(KW)/1
  Product2/1 -> Sum/2
  velocity2distance/1 -> meter2mile/1
  Tractive Energy(KWH)/1 -> Bus Creator/2
  "   acc2velocity"/1 -> velocity2distance/1, Product/2, metrps2mileph/1, Scope4/1
  "Force2acceleration   "/1 -> "   acc2velocity"/1
  Bus Creator/1 -> Bus Selector/1
  Tractive Power(KW)/1 -> Bus Creator/1
  metrps2mileph/1 -> Bus Creator/6, mph to meterps/1, Scope1/1  "Actual vehicle speed(mph)"
  Propeller Energy(J)/1 -> Bus Creator/4
  meter2mile/1 -> Bus Creator/7
  Bus Selector/1 -> Scope3/1, <Actual vehicle speed(mph)>/1  "<Actual vehicle speed(mph)>"
  Magnitude Squared/1 -> Product2/1
  net_tractive_force/1 -> Sum/1, Product/1, Scope/1
  mph to meterps/1 -> Magnitude Squared/1
  Sum/1 -> Scope2/1, "Force2acceleration   "/1
  0.5*Air_density*Drag_coefficient*Frontal_Area/1 -> Product2/2
  Constant2/1 -> Saturation/1
  Constant1/1 -> Sum/3
  Saturation/1 -> Sum/4
